simulink model "model_2"  (R2018b)
settings: Solver=FixedStepAuto  StartTime=0.0  StopTime=100  FixedStep=0.0001  MinStep=0.00001  RelTol=1e-5  AbsTol=1e-5
values from neighbouring files (symbols this model uses):
  m = 1    [Drive.m]    (also in on.m)
  N = 1 / T_f    (= 12.8205128205)    [regler.m]
undefined symbols (not defined in the file or in its folder): X, Y, Z
libraries: sm_lib x72, nesl_utility x28, simulink x5, Contact_Forces_Lib x4, simulink_extras x3, vrlib x1
(part 1 of 3)
settings Model: Creator=Crimson  LastModifiedBy=chjal
settings DataIOCC: LimitDataPoints=on
settings OptimizationCC: LifeSpan=inf
settings DebuggingCC: AlgebraicLoopMsg=none  UnconnectedInputMsg=none  UnconnectedOutputMsg=none  UnconnectedLineMsg=none  AllowSymbolicDim=off  SFUnexpectedBacktrackingDiag=warning  SFNoUnconditionalDefaultTransitionDiag=warning  SFExecutionAtInitializationDiag=none
settings SFSimCC: SimUseLocalCustomCode=off
settings RTWCC: RTWUseLocalCustomCode=off
settings CodeAppCC: StateflowObjectComments=on
settings GRTTargetCC: TargetLangStandard=C89/C90 (ANSI)  GeneratePreprocessorConditionals=Disable all
settings ConfigComp: CovMetricSettings=dw  CovHtmlReporting=on  CovSaveCumulativeToWorkspaceVar=on  CovSaveSingleToWorkspaceVar=on  CovExternalEMLEnable=off  CovSFcnEnable=off
settings SimscapeCC: SimscapeNominalValues="[{\"value\":\"10\",\"unit\":\"V\"},{\"value\":\"1\",\"unit\":\"A\"},{\"value\":\"10\",\"unit\":\"N*m\"},{\"value\":\"10\",\"unit\":\"bar\"},{\"value\":\"100\",\"unit\":\"kJ/kg\"},{\"value\":\"1\",\"unit\":\"kW\"},{\"value\":\"300\",\"unit\":\"K\"},{\"value\":\"100\",\"unit\":\"cm^3/s\"},{\"value\":\"1\",\"unit\":\"kN\"},{\"value\":\"1\",\"unit\":\"g/cm^3\"},{\"value\":\"1\",\"unit\":\"l\"},{\"value\":\"1\",\"unit\":\"cm^2\"},{\"value\":\"60\",\"unit\":\"Hz\"}]"  SimscapeLogType=all  SimscapeLogDataHistory=10000
settings ConfigurationSet: Description=SimMechanics 2G
settings DiagnosticsConfigSet: SimMechanicsRigidlyBoundBlock=none

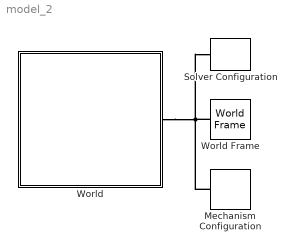
== system model_2 ==
  Mechanism Configuration : sm_lib/Utilities/Mechanism Configuration  UniformGravity=Constant  GravityVector=[0 0 -9.80665]  GravityUnits=m/s^2  LinearizationDelta=0.001
  Solver Configuration : nesl_utility/Solver Configuration  PhysicalDomain=network_engine_domain  SubClassName=solver  LeftPortType=input  RightPortType=generic  Tones=[]  Harmonics=[]  SimulateNoise=off  Profile=off  UseLocalSampling=off  EnableSwitchedLinearOptims=on  FrequencyDomain=off  UseCCode=off  RelTol=0.001  AbsTol=1e-06  MinStep=1e-09  ToWorkspace=off  RevertToSquareIcSolve=off  NumHomotopyIterations=100  PhasorMode=off  PhasorModeNumHarmonics=1  DoDC=off  ResidualTolerance=1e-09  UseLocalSolver=off  LocalSolverChoice=NE_BACKWARD_EULER_ADVANCER  LocalSolverSampleTime=0.001  DoFixedCost=off  MaxNonlinIter=3  MaxModeIter=2  LinearAlgebra=Sparse  EquationFormulation=NE_TIME_EF  DelaysMemoryBudget=1024  AutomaticFiltering=on  FilteringTimeConstant=0.001  PartitionStorageMethod=AS_NEEDED  PartitionMemoryBudget=1024
  World : Subsystem  mask{floorSize=2.5, pathWay=0.5*[-1+0 0-(-3+0.25*tan(2*pi/6)+tan(1*pi/12)+0.5*tan(2*pi/6)); -1+0.5 0-(-3+0.25*tan(2*pi/6)+tan(1*pi/12)+0.5*tan(2*pi/6)); -1+0.5 0.5-(-3+0.25*tan(2*pi/6)+tan(1*pi/12)+0.5*tan(2*pi/6)); -1+1.5 -0.5-(-3+0.25*tan(2*pi/6)+tan(1*pi/12)+0.5*tan(2*pi/6)); -1+1.5 0-(-3+0.25*tan(2*pi/6)+tan(1*pi/12)+0.5*tan(2*pi/6)); -1+2 0-(-3+0.25*tan(2*pi/6)+tan(1*pi/12)+0.5*tan(2*pi/6)); -1+2+cos(5*pi/12) -1+sin(5*pi/12)-(-3+0.25*tan(2*pi/6)+tan(1*pi/12)+0.5*tan(2*pi/6)); -1+2+cos(4*pi/12) -1+sin(4*pi/12)-(-3+0.25*tan(2*pi/6)+tan(1*pi/12)+0.5*tan(2*pi/6)); -1+2+cos(3*pi/12) -1+sin(3*pi/12)-(-3+0.25*tan(2*pi/6)+tan(1*pi/12)+0.5*tan(2*pi/6)); -1+2+cos(2*pi/12) -1+sin(2*pi/12)-(-3+0.25*tan(2*pi/6)+tan(1*pi/12)+0.5*tan(2*pi/6)); -1+2+cos(1*pi/12) -1+sin(1*pi/12)-(-3+0.25*tan(2*pi/6)+tan(1*pi/12)+0.5*tan(2*pi/6)); -1+3 -1-(-3+0.25*tan(2*pi/6)+tan(1*pi/12)+0.5*tan(2*pi/6)); -1+3 -1.5-(-3+0.25*tan(2*pi/6)+tan(1*pi/12)+0.5*tan(2*pi/6)); -1+2.5 -1.75-(-3+0.25*tan(2*pi/6)+tan(1*pi/12)+0.5*tan(2*pi/6)); -1+3.5 -2.25-(-3+0.25*tan(2*pi/6)+tan(1*pi/12)+0.5*tan(2*pi/6)); -1+3 -2.5-(-3+0.25*tan(2*pi/6)+tan(1*pi/12)+0.5*tan(2*pi/6)); -1+3 -3-(-3+0.25*tan(2*pi/6)+tan(1*pi/12)+0.5*tan(2*pi/6)); -1+2.75 -3+0.25*tan(2*pi/6)-(-3+0.25*tan(2*pi/6)+tan(1*pi/12)+0.5*tan(2*pi/6)); -1+0.75 -3+0.25*tan(2*pi/6)-(-3+0.25*tan(2*pi/6)+tan(1*pi/12)+0.5*tan(2*pi/6)); -1+1.75 -3+0.25*tan(2*pi/6)+tan(1*pi/12)-(-3+0.25*tan(2*pi/6)+tan(1*pi/12)+0.5*tan(2*pi/6)); -1+1.25 -3+0.25*tan(2*pi/6)+tan(1*pi/12)+0.5*tan(2*pi/6)-(-3+0.25*tan(2*pi/6)+tan(1*pi/12)+0.5*tan(2*pi/6)); -1+0 -3+0.25*tan(2*pi/6)+tan(1*pi/12)+0.5*tan(2*pi/6)-(-3+0.25*tan(2*pi/6)+tan(1*pi/12)+0.5*tan(2*pi/6)); -1+0 0-(-3+0.25*tan(2*pi/6)+tan(1*pi/12)+0.5*tan(2*pi/6))], floorColor=[1.0 1.0 1.0], floorStiffness=7500, floorDamping=50}
  World Frame : sm_lib/Frames and Transforms/World Frame
  connections:
  Mechanism Configuration/RConn1 -- World/RConn1 -- Solver Configuration/RConn1 -- World Frame/RConn1

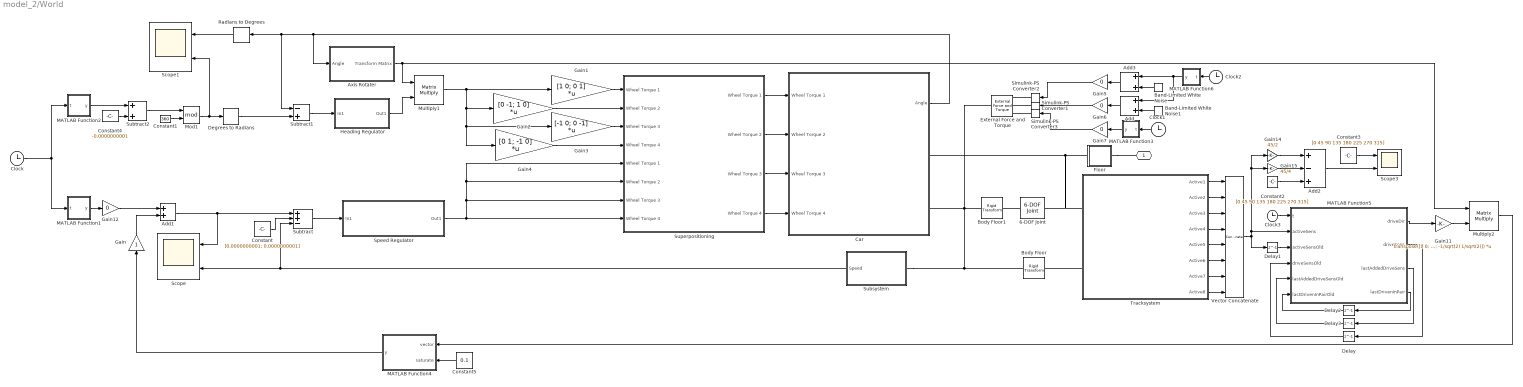
== system model_2/World ==
  6-DOF Joint : sm_lib/Joints/6-DOF Joint  SenseConstraintForce=off  SenseConstraintForceX=off  SenseConstraintForceY=off  SenseConstraintForceZ=off  SenseConstraintTorque=off  SenseConstraintTorqueX=off  SenseConstraintTorqueY=off  SenseConstraintTorqueZ=off  SenseTotalForce=off  SenseTotalForceX=off  SenseTotalForceY=off  SenseTotalForceZ=off  SenseTotalTorque=off  SenseTotalTorqueX=off  SenseTotalTorqueY=off  SenseTotalTorqueZ=off  CompositeWrenchDir=FollowerOnBase  CompositeWrenchFrame=BaseFrame  PxEquilibriumPosition=0  PxEquilibriumPositionUnits=m  PxSpringStiffness=0  PxSpringStiffnessUnits=N/m  PxDampingCoefficient=0  PxDampingCoefficientUnits=N/(m/s)  PxTorqueActuationMode=NoTorque  PxMotionActuationMode=ComputedMotion  PxSensePosition=off  PxSenseVelocity=off  PxSenseAcceleration=off  PxSenseTorqueForce=off  PxPositionTargetSpecify=off  PxPositionTargetPriority=High  PxPositionTargetValue=0  PxPositionTargetValueUnits=m  PxVelocityTargetSpecify=off  PxVelocityTargetPriority=High  PxVelocityTargetValue=0  PxVelocityTargetValueUnits=m/s  PyEquilibriumPosition=0  PyEquilibriumPositionUnits=m  PySpringStiffness=0  PySpringStiffnessUnits=N/m  PyDampingCoefficient=0  PyDampingCoefficientUnits=N/(m/s)  PyTorqueActuationMode=NoTorque  PyMotionActuationMode=ComputedMotion  PySensePosition=off  PySenseVelocity=off  PySenseAcceleration=off  PySenseTorqueForce=off  PyPositionTargetSpecify=off  PyPositionTargetPriority=High  PyPositionTargetValue=0  PyPositionTargetValueUnits=m  PyVelocityTargetSpecify=off  PyVelocityTargetPriority=High  PyVelocityTargetValue=0  PyVelocityTargetValueUnits=m/s  PzEquilibriumPosition=0  PzEquilibriumPositionUnits=m  PzSpringStiffness=0  PzSpringStiffnessUnits=N/m  PzDampingCoefficient=0  PzDampingCoefficientUnits=N/(m/s)  PzTorqueActuationMode=NoTorque  PzMotionActuationMode=ComputedMotion  PzSensePosition=off  PzSenseVelocity=off  PzSenseAcceleration=off  PzSenseTorqueForce=off  PzPositionTargetSpecify=off  PzPositionTargetPriority=High  PzPositionTargetValue=0  PzPositionTargetValueUnits=m  PzVelocityTargetSpecify=off  PzVelocityTargetPriority=High  PzVelocityTargetValue=0  PzVelocityTargetValueUnits=m/s  SphDefPosRotationMethod=None  SphDefPosRotationAngleUnits=deg  SphDefPosRotationStandardAxis=+Z  SphDefPosRotationAngle=0.0  SphDefPosRotationArbitraryAxis=[0 0 1]  SphDefPosFollAlignAxisA=+X  SphDefPosBaseAlignAxisA=+Y  SphDefPosFollAlignAxisB=+Y  SphDefPosBaseAlignAxisB=+Z  SphDefPosRotationSequenceAxes=FollowerAxes  SphDefPosRotationSequence=XYX  SphDefPosRotationSequenceAngles=[0 0 0]  SphDefPosRotationSequenceAnglesUnits=deg  SphDefPosRotationMatrix=[1 0 0; 0 1 0; 0 0 1]  SphEqPosRotationMethod=None  SphEqPosRotationAngleUnits=deg  SphEqPosRotationStandardAxis=+Z  SphEqPosRotationAngle=0.0  SphEqPosRotationArbitraryAxis=[0 0 1]  SphEqPosFollAlignAxisA=+X  SphEqPosBaseAlignAxisA=+Y  SphEqPosFollAlignAxisB=+Y  SphEqPosBaseAlignAxisB=+Z  SphEqPosRotationSequenceAxes=FollowerAxes  SphEqPosRotationSequence=XYX  SphEqPosRotationSequenceAngles=[0 0 0]  SphEqPosRotationSequenceAnglesUnits=deg  SphEqPosRotationMatrix=[1 0 0; 0 1 0; 0 0 1]  SphSpringStiffness=0  SphSpringStiffnessUnits=N*m/deg  SphDampingCoefficient=0  SphDampingCoefficientUnits=N*m/(deg/s)  SphActuateTorqueX=off  SphActuateTorqueY=off  SphActuateTorqueZ=off  SphActuateTorque=off  SphTorqueActuationMode=NoTorque  SphMotionActuationMode=ComputedMotion  SphActuationFrame=BaseFrame  SphSensePosition=off  SphSenseVelocityX=off  SphSenseVelocityY=off  SphSenseVelocityZ=off  SphSenseVelocity=off  SphSenseAccelerationX=off  SphSenseAccelerationY=off  SphSenseAccelerationZ=off  SphSenseAcceleration=off  SphSenseTorqueX=off  SphSenseTorqueY=off  SphSenseTorqueZ=off  SphSenseTorqueForce=off  SphSensingFrame=BaseFrame  SphPositionTargetRotationMethod=None  SphPositionTargetRotationAngleUnits=deg  SphPositionTargetRotationStandardAxis=+Z  SphPositionTargetRotationAngle=0.0  SphPositionTargetRotationArbitraryAxis=[0 0 1]  SphPositionTargetFollAlignAxisA=+X  SphPositionTargetBaseAlignAxisA=+Y  SphPositionTargetFollAlignAxisB=+Y  SphPositionTargetBaseAlignAxisB=+Z  SphPositionTargetRotationSequenceAxes=FollowerAxes  SphPositionTargetRotationSequence=XYX  SphPositionTargetRotationSequenceAngles=[0 0 0]  SphPositionTargetRotationSequenceAnglesUnits=deg  SphPositionTargetRotationMatrix=[1 0 0; 0 1 0; 0 0 1]  SphPositionTargetSpecify=off  SphPositionTargetPriority=High  SphVelocityTargetValue=[0 0 0]  SphVelocityTargetValueUnits=deg/s  SphVelocityTargetSpecify=off  SphVelocityTargetPriority=High  SphVelocityTargetInFollowerFrame=on
  Add : Sum
  Add1 : Sum
  Add2 : Sum  Inputs=+-+
  Add3 : Sum
  Axis Rotater : Subsystem
  Band-Limited White Noise : simulink/Sources/Band-Limited White Noise  Cov=[0.001]  Ts=0.1  seed=[23341]
  Band-Limited White Noise1 : simulink/Sources/Band-Limited White Noise  Cov=[0.001]  Ts=0.1  seed=[23342]
  Body Floor : sm_lib/Frames and Transforms/Rigid Transform  TranslationMethod=None  TranslationStandardOffset=1  TranslationLengthUnit=m  TranslationStandardAxis=-Z  TranslationCartesianOffset=[0 0 0]  TranslationROffset=0  TranslationROffsetUnits=m  TranslationZOffset=0  TranslationZOffsetUnits=m  TranslationThetaOffset=0  TranslationThetaOffsetUnits=deg  RotationMethod=None  RotationAngleUnits=deg  RotationStandardAxis=-Z  RotationAngle=90  RotationArbitraryAxis=[0 0 1]  FollAlignAxisA=+X  BaseAlignAxisA=+Y  FollAlignAxisB=+Y  BaseAlignAxisB=+Z  RotationSequenceAxes=FollowerAxes  RotationSequence=XYX  RotationSequenceAngles=[0 0 0]  RotationSequenceAnglesUnits=deg  RotationMatrix=[1 0 0; 0 1 0; 0 0 1]
  Body Floor1 : sm_lib/Frames and Transforms/Rigid Transform  TranslationMethod=StandardAxis  TranslationStandardOffset=0.25  TranslationLengthUnit=m  TranslationStandardAxis=+X  TranslationCartesianOffset=[0 0 0]  TranslationROffset=0  TranslationROffsetUnits=m  TranslationZOffset=0  TranslationZOffsetUnits=m  TranslationThetaOffset=0  TranslationThetaOffsetUnits=deg  RotationMethod=None  RotationAngleUnits=deg  RotationStandardAxis=-Z  RotationAngle=90  RotationArbitraryAxis=[0 0 1]  FollAlignAxisA=+X  BaseAlignAxisA=+Y  FollAlignAxisB=+Y  BaseAlignAxisB=+Z  RotationSequenceAxes=FollowerAxes  RotationSequence=XYX  RotationSequenceAngles=[0 0 0]  RotationSequenceAnglesUnits=deg  RotationMatrix=[1 0 0; 0 1 0; 0 0 1]
  Car : Subsystem  mask{wheelLengthOffset=120/1000, wheelWidthOffset=100/1000, radius=73/2/1000, angle=0}
  Clock{,1..3} (4 alike) : Clock
  Constant : Constant  Value=[0.0000000001; 0.0000000001]
  Constant1 : Constant  Value=360
  Constant2 : Constant  Value=[0 45 90 135 180 225 270 315]
  Constant3 : Constant  Value=[0 45 90 135 180 225 270 315]
  Constant4 : Constant  Value=-0.0000000001
  Constant5 : Constant  Value=0.1
  Degrees to Radians : simulink_extras/Transformations/Degrees to Radians
  Delay : Delay  DelayLength=1  InitialCondition=[0,0,0,0,1,0,0,0]
  Delay1 : Delay  DelayLength=1  InitialCondition=[1,1,1,1,1,1,1,1]
  Delay2 : Delay  DelayLength=1  InitialCondition=[1,0,0,0,0,0,0,0]
  Delay3 : Delay  DelayLength=1  InitialCondition=[1,0,1,0]
  External Force and Torque : sm_lib/Forces and Torques/External Force and Torque  ForceResolutionFrame=World  EnableForceX=on  EnableForceY=on  EnableForceZ=off  EnableForce=off  TorqueResolutionFrame=World  EnableTorqueX=off  EnableTorqueY=off  EnableTorqueZ=on  EnableTorque=off
  Floor : Subsystem
  Gain : Gain
  Gain1 : Gain  Gain=[1 0; 0 1]  Multiplication=Matrix(K*u)
  Gain11 : Gain  Gain=transpose([1 0; 1/sqrt(2) 1/sqrt(2); 0 1; -1/sqrt(2) 1/sqrt(2)])  Multiplication=Matrix(K*u)
  Gain{5..7,12} (4 alike) : Gain  Gain=0
  Gain14 : Gain  Gain=45/2
  Gain15 : Gain  Gain=45/4
  Gain2 : Gain  Gain=[0 -1; 1 0]  Multiplication=Matrix(K*u)
  Gain3 : Gain  Gain=[-1 0; 0 -1]  Multiplication=Matrix(K*u)
  Gain4 : Gain  Gain=[0 1; -1 0]  Multiplication=Matrix(K*u)
  Heading Regulator : Subsystem
  MATLAB Function1 : MATLAB Function  TreatAsAtomicUnit=on
  MATLAB Function2 : MATLAB Function  TreatAsAtomicUnit=on
  MATLAB Function3 : MATLAB Function  TreatAsAtomicUnit=on
  MATLAB Function4 : MATLAB Function  TreatAsAtomicUnit=on
  MATLAB Function5 : MATLAB Function  TreatAsAtomicUnit=on
  MATLAB Function6 : MATLAB Function  TreatAsAtomicUnit=on
  Mod1 : Math  Operator=mod  SaturateOnIntegerOverflow=on
  Multiply1 : Product  Multiplication=Matrix(*)
  Multiply2 : Product  Multiplication=Matrix(*)
  Radians to Degrees : simulink_extras/Transformations/Radians to Degrees
  Scope : Scope  NumInputPorts=2
  Scope1 : Scope  NumInputPorts=2
  Scope3 : Scope  NumInputPorts=2
  Simulink-PS Converter1 : nesl_utility/Simulink-PS Converter  PhysicalDomain=network_engine_domain  SubClassName=ps_input  LeftPortType=input  RightPortType=output  PseudoPeriodic=off  Frequencies=[]  NoiseDistribution=none  NoiseParameters=[]  Unit=N  AffineConversion=off  FilteringAndDerivatives=provide  SimscapeFilterOrder=1  InputFilterTimeConstant=0.001  UdotUserProvided=0
  Simulink-PS Converter2 : nesl_utility/Simulink-PS Converter  PhysicalDomain=network_engine_domain  SubClassName=ps_input  LeftPortType=input  RightPortType=output  PseudoPeriodic=off  Frequencies=[]  NoiseDistribution=none  NoiseParameters=[]  Unit=N  AffineConversion=off  FilteringAndDerivatives=provide  SimscapeFilterOrder=1  InputFilterTimeConstant=0.001  UdotUserProvided=0
  Simulink-PS Converter3 : nesl_utility/Simulink-PS Converter  PhysicalDomain=network_engine_domain  SubClassName=ps_input  LeftPortType=input  RightPortType=output  PseudoPeriodic=off  Frequencies=[]  NoiseDistribution=none  NoiseParameters=[]  Unit=N*m  AffineConversion=off  FilteringAndDerivatives=provide  SimscapeFilterOrder=1  InputFilterTimeConstant=0.001  UdotUserProvided=0
  Speed Regulator : Subsystem
  Subsystem : Subsystem
  Subtract : Sum  Inputs=++-
  Subtract1 : Sum  Inputs=-+
  Subtract2 : Sum
  Superpositioning : Subsystem
  Tracksystem : Subsystem  InitFcn=run bana2  mask{thickness=50/2000, linePath=0.5*[-1.5+0 0-(-3+0.25*tan(2*pi/6)+tan(1*pi/12)+0.5*tan(2*pi/6)); -1.5+0 -3+0.25*tan(2*pi/6)+tan(1*pi/12)+0.5*tan(2*pi/6)-(-3+0.25*tan(2*pi/6)+tan(1*pi/12)+0.5*tan(2*pi/6)); -1.5+1.25 -3+0.25*tan(2*pi/6)+tan(1*pi/12)+0.5*tan(2*pi/6)-(-3+0.25*tan(2*pi/6)+tan(1*pi/12)+0.5*tan(2*pi/6)); -1.5+1.75 -3+0.25*tan(2*pi/6)+tan(1*pi/12)-(-3+0.25*tan(2*pi/6)+tan(1*pi/12)+0.5*tan(2*pi/6)); -1.5+0.75 -3+0.25*tan(2*pi/6)-(-3+0.25*tan(2*pi/6)+tan(1*pi/12)+0.5*tan(2*pi/6)); -1.5+2.75 -3+0.25*tan(2*pi/6)-(-3+0.25*tan(2*pi/6)+tan(1*pi/12)+0.5*tan(2*pi/6)); -1.5+3 -3-(-3+0.25*tan(2*pi/6)+tan(1*pi/12)+0.5*tan(2*pi/6)); -1.5+3 -2.5-(-3+0.25*tan(2*pi/6)+tan(1*pi/12)+0.5*tan(2*pi/6)); -1.5+3.5 -2.25-(-3+0.25*tan(2*pi/6)+tan(1*pi/12)+0.5*tan(2*pi/6)); -1.5+2.5 -1.75-(-3+0.25*tan(2*pi/6)+tan(1*pi/12)+0.5*tan(2*pi/6)); -1.5+3 -1.5-(-3+0.25*tan(2*pi/6)+tan(1*pi/12)+0.5*tan(2*pi/6)); -1.5+3 -1-(-3+0.25*tan(2*pi/6)+tan(1*pi/12)+0.5*tan(2*pi/6)); -1.5+2+cos(1*pi/12) -1+sin(1*pi/12)-(-3+0.25*tan(2*pi/6)+tan(1*pi/12)+0.5*tan(2*pi/6)); -1.5+2+cos(2*pi/12) -1+sin(2*pi/12)-(-3+0.25*tan(2*pi/6)+tan(1*pi/12)+0.5*tan(2*pi/6)); -1.5+2+cos(3*pi/12) -1+sin(3*pi/12)-(-3+0.25*tan(2*pi/6)+tan(1*pi/12)+0.5*tan(2*pi/6)); -1.5+2+cos(4*pi/12) -1+sin(4*pi/12)-(-3+0.25*tan(2*pi/6)+tan(1*pi/12)+0.5*tan(2*pi/6)); -1.5+2+cos(5*pi/12) -1+sin(5*pi/12)-(-3+0.25*tan(2*pi/6)+tan(1*pi/12)+0.5*tan(2*pi/6)); -1.5+2 0-(-3+0.25*tan(2*pi/6)+tan(1*pi/12)+0.5*tan(2*pi/6)); -1.5+1.5 0-(-3+0.25*tan(2*pi/6)+tan(1*pi/12)+0.5*tan(2*pi/6)); -1.5+1.5 -0.5-(-3+0.25*tan(2*pi/6)+tan(1*pi/12)+0.5*tan(2*pi/6)); -1.5+0.5 0.5-(-3+0.25*tan(2*pi/6)+tan(1*pi/12)+0.5*tan(2*pi/6)); -1.5+0.5 0-(-3+0.25*tan(2*pi/6)+tan(1*pi/12)+0.5*tan(2*pi/6)); -1.5+0 0-(-3+0.25*tan(2*pi/6)+tan(1*pi/12)+0.5*tan(2*pi/6))];, sensorLength=28/1000, sensorWidth=10/1000, sensorHeight=10/1000, sensorRadius=50/1000, sensorSize=5/1000}
      mask prompts: sensorSize "sensorSize (debugging only)"
  Vector Concatenate : Concatenate  NumInputs=8
  " " : PMIOPort  Side=Right
  wires:
  Mod1/1 -> Degrees to Radians/1, Scope1/2
  Constant1/1 -> Mod1/2
  Car/1(Angle) -> Axis Rotater/1(Angle), Radians to Degrees/1, Subtract1/1
  Gain1/1 -> Superpositioning/1(Wheel Torque 1)
  Gain2/1 -> Superpositioning/2(Wheel Torque 2)
  Gain3/1 -> Superpositioning/3(Wheel Torque 3)
  Gain4/1 -> Superpositioning/4(Wheel Torque 4)
  Multiply1/1 -> Gain2/1, Gain4/1, Gain3/1, Gain1/1
  Subtract/1 -> Speed Regulator/1(In1)
  Axis Rotater/1(Transform Matrix) -> Multiply1/1, Multiply2/1
  Subtract1/1 -> Heading Regulator/1(In1)
  Heading Regulator/1(Out1) -> Multiply1/2
  Degrees to Radians/1 -> Subtract1/2
  Radians to Degrees/1 -> Scope1/1
  Constant/1 -> Subtract/2
  MATLAB Function1/1(y) -> Gain12/1
  Gain12/1 -> Add1/1
  MATLAB Function4/1(y) -> Gain/1
  Tracksystem/1(Active1) -> Vector Concatenate/1
  Tracksystem/2(Active2) -> Vector Concatenate/2
  Tracksystem/3(Active3) -> Vector Concatenate/3
  Tracksystem/4(Active4) -> Vector Concatenate/4
  Tracksystem/5(Active5) -> Vector Concatenate/5
  Tracksystem/6(Active6) -> Vector Concatenate/6
  Tracksystem/7(Active7) -> Vector Concatenate/7
  Tracksystem/8(Active8) -> Vector Concatenate/8
  Gain14/1 -> Add2/1
  Constant3/1 -> Scope3/1
  Add2/1 -> Scope3/2
  Constant2/1 -> Add2/3
  Gain15/1 -> Add2/2
  Superpositioning/3(" Wheel Torque 3") -> Car/3(Wheel Torque 3)
  Superpositioning/4(" Wheel Torque 4") -> Car/4(Wheel Torque 4)
  Subtract2/1 -> Mod1/1
  Constant4/1 -> Subtract2/2
  MATLAB Function2/1(y) -> Subtract2/1
  Speed Regulator/1(Out1) -> Superpositioning/5("Wheel Torque 1 "), Superpositioning/6("Wheel Torque 2 "), Superpositioning/7("Wheel Torque 3 "), Superpositioning/8("Wheel Torque 4 ")
  Gain11/1 -> Multiply2/2
  Multiply2/1 -> MATLAB Function4/1(vector)
  Constant5/1 -> MATLAB Function4/2(saturate)
  Vector Concatenate/1 -> MATLAB Function5/2(activeSens), Gain14/1, Gain15/1, Delay1/1
  Delay/1 -> MATLAB Function5/4(driveSensOld)
  MATLAB Function5/1(driveDir) -> Gain11/1
  MATLAB Function5/2(driveSens) -> Delay/1
  Delay1/1 -> MATLAB Function5/3(activeSensOld)
  Add1/1 -> Scope/1, Subtract/1
  Subsystem/1(Speed) -> Scope/2, Subtract/3
  MATLAB Function5/3(lastAddedDriveSens) -> Delay3/1
  Delay3/1 -> MATLAB Function5/5(lastAddedDriveSensOld)
  Gain/1 -> Add1/2
  Superpositioning/2(" Wheel Torque 2") -> Car/2(Wheel Torque 2)
  Clock1/1 -> MATLAB Function3/1(t)
  Gain5/1 -> Simulink-PS Converter2/1
  Gain6/1 -> Simulink-PS Converter1/1
  Gain7/1 -> Simulink-PS Converter3/1
  Clock2/1 -> MATLAB Function6/1(t)
  Clock3/1 -> MATLAB Function5/1(t)
  Clock/1 -> MATLAB Function1/1(t), MATLAB Function2/1(t)
  Add/1 -> Gain6/1
  Add3/1 -> Gain5/1
  MATLAB Function6/1(y) -> Add3/1, Add/1
  Band-Limited White Noise/1 -> Add3/2
  Band-Limited White Noise1/1 -> Add/2
  MATLAB Function3/1(y) -> Gain7/1
  Superpositioning/1(" Wheel Torque 1") -> Car/1(Wheel Torque 1)
  MATLAB Function5/4(lastDrivenInPair) -> Delay2/1
  Delay2/1 -> MATLAB Function5/6(lastDrivenInPairOld)
  connections:
  Floor/RConn1 -- " "/RConn1
  Floor/LConn1 -- Tracksystem/LConn1 -- 6-DOF Joint/RConn1 -- Car/RConn1
  Subsystem/LConn1 -- Body Floor/RConn1 -- Car/RConn2 -- Body Floor1/LConn1 -- External Force and Torque/RConn1
  Tracksystem/LConn2 -- Body Floor/LConn1
  Simulink-PS Converter2/RConn1 -- External Force and Torque/LConn1
  Simulink-PS Converter1/RConn1 -- External Force and Torque/LConn2
  Simulink-PS Converter3/RConn1 -- External Force and Torque/LConn3
  6-DOF Joint/LConn1 -- Body Floor1/RConn1

== system model_2/World/Axis Rotater ==
  Angle : Inport
  MATLAB Function : MATLAB Function  TreatAsAtomicUnit=on
  Transform Matrix : Outport
  wires:
  Angle/1 -> MATLAB Function/1(u)
  MATLAB Function/1(y) -> Transform Matrix/1

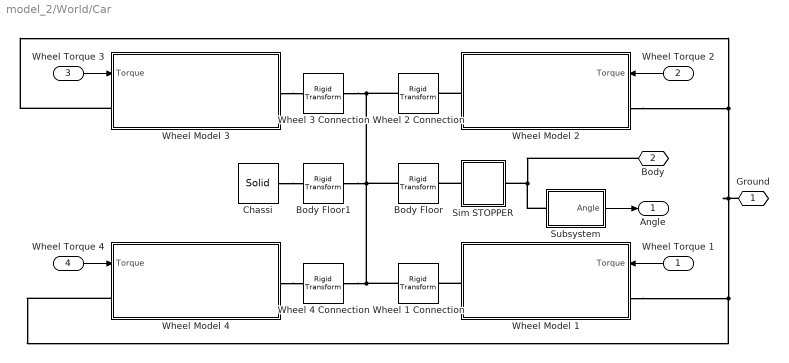
== system model_2/World/Car ==
  Wheel Torque 1 : Inport
  Wheel Torque 2 : Inport  Port=2
  Wheel Torque 3 : Inport  Port=3
  Wheel Torque 4 : Inport  Port=4
  Body Floor : sm_lib/Frames and Transforms/Rigid Transform  TranslationMethod=StandardAxis  TranslationStandardOffset=radius-4.8*10^-4  TranslationLengthUnit=m  TranslationStandardAxis=-Z  TranslationCartesianOffset=[0 0 0]  TranslationROffset=0  TranslationROffsetUnits=m  TranslationZOffset=0  TranslationZOffsetUnits=m  TranslationThetaOffset=0  TranslationThetaOffsetUnits=deg  RotationMethod=StandardAxis  RotationAngleUnits=deg  RotationStandardAxis=-Z  RotationAngle=angle  RotationArbitraryAxis=[0 0 1]  FollAlignAxisA=+X  BaseAlignAxisA=+Y  FollAlignAxisB=+Y  BaseAlignAxisB=+Z  RotationSequenceAxes=FollowerAxes  RotationSequence=XYX  RotationSequenceAngles=[0 0 0]  RotationSequenceAnglesUnits=deg  RotationMatrix=[1 0 0; 0 1 0; 0 0 1]
  Body Floor1 : sm_lib/Frames and Transforms/Rigid Transform  TranslationMethod=Cartesian  TranslationStandardOffset=0  TranslationLengthUnit=m  TranslationStandardAxis=-Z  TranslationCartesianOffset=[wheelLengthOffset wheelWidthOffset 0]  TranslationROffset=0  TranslationROffsetUnits=m  TranslationZOffset=0  TranslationZOffsetUnits=m  TranslationThetaOffset=0  TranslationThetaOffsetUnits=deg  RotationMethod=None  RotationAngleUnits=deg  RotationStandardAxis=+Z  RotationAngle=0.0  RotationArbitraryAxis=[0 0 1]  FollAlignAxisA=+X  BaseAlignAxisA=+Y  FollAlignAxisB=+Y  BaseAlignAxisB=+Z  RotationSequenceAxes=FollowerAxes  RotationSequence=XYX  RotationSequenceAngles=[0 0 0]  RotationSequenceAnglesUnits=deg  RotationMatrix=[1 0 0; 0 1 0; 0 0 1]
  Chassi : sm_lib/Body Elements/Solid  InertiaType=CalculateFromGeometry  Mass=1  MassUnits=kg  CenterOfMass=[0 0 0]  CenterOfMassUnits=m  MomentsOfInertia=[1 1 1]  MomentsOfInertiaUnits=kg*m^2  ProductsOfInertia=[0 0 0]  ProductsOfInertiaUnits=kg*m^2  BasedOnType=Density  Density=2700  DensityUnits=kg/m^3  DoExposeReferenceFrame=on  SerializedFrames=<Frames/>  GraphicType=FromGeometry  MarkerShape=Sphere  MarkerSize=10  GraphicVisPropType=SimpleVisualProperties  GraphicDiffuseColor=[0.6 0.8 1.0]  GraphicSpecularColor=[0.5 0.5 0.5 1.0]  GraphicAmbientColor=[0.15 0.15 0.15 1.0]  GraphicEmissiveColor=[0.0 0.0 0.0 1.0]  GraphicShininess=75  GraphicOpacity=0.5  GeometryShape=FromFile  RectangleSize=[1 1]  RectangleSizeUnits=m  BrickDimensions=[1 1 1]  BrickDimensionUnits=m  CylinderRadius=1  CylinderRadiusUnits=m  CylinderLength=1  CylinderLengthUnits=m  SphereRadius=1  SphereRadiusUnits=m  EllipsoidRadii=[1 1 .5]  EllipsoidRadiiUnits=m  ExtrusionCrossSection=[1 1; -1 1; -1 -1; 1 -1]  ExtrusionCrossSectionUnits=m  ExtrusionLength=1  ExtrusionLengthUnits=m  PolygonNumSides=3  PolygonOuterRadius=1  PolygonOuterRadiusUnits=m  ExtGeomFileType=STEP  ExtGeomFileName=bas.stp  ExtGeomFileUnits=m  RevolutionCrossSection=[1 1; 1 -1; 2 -1; 2 1]  RevolutionCrossSectionUnits=m  RevolutionExtent=Custom  RevolutionAngle=180  RevolutionAngleUnits=deg
  Sim STOPPER : Subsystem
  Subsystem : Subsystem
  Wheel 1 Connection : sm_lib/Frames and Transforms/Rigid Transform  TranslationMethod=Cartesian  TranslationStandardOffset=1  TranslationLengthUnit=m  TranslationStandardAxis=-Z  TranslationCartesianOffset=[wheelLengthOffset -wheelWidthOffset 0]  TranslationROffset=0  TranslationROffsetUnits=m  TranslationZOffset=0  TranslationZOffsetUnits=m  TranslationThetaOffset=0  TranslationThetaOffsetUnits=deg  RotationMethod=StandardAxis  RotationAngleUnits=deg  RotationStandardAxis=+Z  RotationAngle=180  RotationArbitraryAxis=[0 0 1]  FollAlignAxisA=+X  BaseAlignAxisA=+Y  FollAlignAxisB=+Y  BaseAlignAxisB=+Z  RotationSequenceAxes=FollowerAxes  RotationSequence=XYX  RotationSequenceAngles=[0 0 0]  RotationSequenceAnglesUnits=deg  RotationMatrix=[1 0 0; 0 1 0; 0 0 1]
  Wheel 2 Connection : sm_lib/Frames and Transforms/Rigid Transform  TranslationMethod=Cartesian  TranslationStandardOffset=0  TranslationLengthUnit=m  TranslationStandardAxis=-Z  TranslationCartesianOffset=[wheelLengthOffset wheelWidthOffset 0]  TranslationROffset=0  TranslationROffsetUnits=m  TranslationZOffset=0  TranslationZOffsetUnits=m  TranslationThetaOffset=0  TranslationThetaOffsetUnits=deg  RotationMethod=StandardAxis  RotationAngleUnits=deg  RotationStandardAxis=+Z  RotationAngle=0.0  RotationArbitraryAxis=[0 0 1]  FollAlignAxisA=+X  BaseAlignAxisA=+Y  FollAlignAxisB=+Y  BaseAlignAxisB=+Z  RotationSequenceAxes=FollowerAxes  RotationSequence=XYX  RotationSequenceAngles=[0 0 0]  RotationSequenceAnglesUnits=deg  RotationMatrix=[1 0 0; 0 1 0; 0 0 1]
  Wheel 3 Connection : sm_lib/Frames and Transforms/Rigid Transform  TranslationMethod=Cartesian  TranslationStandardOffset=0  TranslationLengthUnit=m  TranslationStandardAxis=-Z  TranslationCartesianOffset=[-wheelLengthOffset wheelWidthOffset 0]  TranslationROffset=0  TranslationROffsetUnits=m  TranslationZOffset=0  TranslationZOffsetUnits=m  TranslationThetaOffset=0  TranslationThetaOffsetUnits=deg  RotationMethod=StandardAxis  RotationAngleUnits=deg  RotationStandardAxis=+Z  RotationAngle=0.0  RotationArbitraryAxis=[0 0 1]  FollAlignAxisA=+X  BaseAlignAxisA=+Y  FollAlignAxisB=+Y  BaseAlignAxisB=+Z  RotationSequenceAxes=FollowerAxes  RotationSequence=XYX  RotationSequenceAngles=[0 0 0]  RotationSequenceAnglesUnits=deg  RotationMatrix=[1 0 0; 0 1 0; 0 0 1]
  Wheel 4 Connection : sm_lib/Frames and Transforms/Rigid Transform  TranslationMethod=Cartesian  TranslationStandardOffset=0  TranslationLengthUnit=m  TranslationStandardAxis=-Z  TranslationCartesianOffset=[-wheelLengthOffset -wheelWidthOffset 0]  TranslationROffset=0  TranslationROffsetUnits=m  TranslationZOffset=0  TranslationZOffsetUnits=m  TranslationThetaOffset=0  TranslationThetaOffsetUnits=deg  RotationMethod=StandardAxis  RotationAngleUnits=deg  RotationStandardAxis=+Z  RotationAngle=180  RotationArbitraryAxis=[0 0 1]  FollAlignAxisA=+X  BaseAlignAxisA=+Y  FollAlignAxisB=+Y  BaseAlignAxisB=+Z  RotationSequenceAxes=FollowerAxes  RotationSequence=XYX  RotationSequenceAngles=[0 0 0]  RotationSequenceAnglesUnits=deg  RotationMatrix=[1 0 0; 0 1 0; 0 0 1]
  Wheel Model 1 : Subsystem
  Wheel Model 2 : Subsystem
  Wheel Model 3 : Subsystem
  Wheel Model 4 : Subsystem
  Ground : PMIOPort  Side=Right
  Body : PMIOPort  Port=2  Side=Right
  Angle : Outport
  wires:
  Wheel Torque 2/1 -> Wheel Model 2/1(Torque)
  Wheel Torque 3/1 -> Wheel Model 3/1(Torque)
  Subsystem/1(Angle) -> Angle/1
  Wheel Torque 1/1 -> Wheel Model 1/1(Torque)
  Wheel Torque 4/1 -> Wheel Model 4/1(Torque)
  connections:
  Wheel 2 Connection/LConn1 -- Wheel 4 Connection/LConn1 -- Wheel 1 Connection/LConn1 -- Body Floor1/RConn1 -- Body Floor/LConn1 -- Wheel 3 Connection/LConn1
  Subsystem/LConn1 -- Body/RConn1 -- Sim STOPPER/RConn1
  Wheel Model 3/RConn1 -- Wheel 3 Connection/RConn1
  Chassi/RConn1 -- Body Floor1/LConn1
  Wheel Model 2/RConn1 -- Wheel 2 Connection/RConn1
  Sim STOPPER/LConn1 -- Body Floor/RConn1
  Ground/RConn1 -- Wheel Model 3/LConn1 -- Wheel Model 2/LConn1 -- Wheel Model 4/LConn1 -- Wheel Model 1/LConn1
  Wheel Model 1/RConn1 -- Wheel 1 Connection/RConn1
  Wheel Model 4/RConn1 -- Wheel 4 Connection/RConn1

== system model_2/World/Floor ==
  Floor : sm_lib/Body Elements/Solid  InertiaType=CalculateFromGeometry  Mass=1  MassUnits=kg  CenterOfMass=[0 0 0]  CenterOfMassUnits=m  MomentsOfInertia=[1 1 1]  MomentsOfInertiaUnits=kg*m^2  ProductsOfInertia=[0 0 0]  ProductsOfInertiaUnits=kg*m^2  BasedOnType=Density  Density=1000  DensityUnits=kg/(m^3)  DoExposeReferenceFrame=on  SerializedFrames=<Frames/>  GraphicType=FromGeometry  MarkerShape=Cube  MarkerSize=5000  GraphicVisPropType=SimpleVisualProperties  GraphicDiffuseColor=floorColor  GraphicSpecularColor=[0.5 0.5 0.5 1.0]  GraphicAmbientColor=[0.15 0.15 0.15 1.0]  GraphicEmissiveColor=[0.0 0.0 0.0 1.0]  GraphicShininess=75  GraphicOpacity=1.0  GeometryShape=Brick  RectangleSize=[1 1]  RectangleSizeUnits=m  BrickDimensions=[floorSize floorSize, floorSize/1000]  BrickDimensionUnits=m  CylinderRadius=1  CylinderRadiusUnits=m  CylinderLength=1  CylinderLengthUnits=m  SphereRadius=1  SphereRadiusUnits=m  EllipsoidRadii=[1 1 1]  EllipsoidRadiiUnits=m  ExtrusionCrossSection=[1 1; -1 1; -1 -1; 1 -1]  ExtrusionCrossSectionUnits=m  ExtrusionLength=floorSize/1000  ExtrusionLengthUnits=m  PolygonNumSides=3  PolygonOuterRadius=1  PolygonOuterRadiusUnits=m  ExtGeomFileType=STL  ExtGeomFileUnits=m  RevolutionCrossSection=[1 1; 1 -1; 2 -1; 2 1]  RevolutionCrossSectionUnits=m  RevolutionExtent=Full  RevolutionAngle=180  RevolutionAngleUnits=deg
  Floor Surface : sm_lib/Frames and Transforms/Rigid Transform  TranslationMethod=StandardAxis  TranslationStandardOffset=floorSize/2000  TranslationLengthUnit=m  TranslationStandardAxis=+Z  TranslationCartesianOffset=[0 0 0]  TranslationROffset=0  TranslationROffsetUnits=m  TranslationZOffset=0  TranslationZOffsetUnits=m  TranslationThetaOffset=0  TranslationThetaOffsetUnits=deg  RotationMethod=None  RotationAngleUnits=deg  RotationStandardAxis=+Z  RotationAngle=0.0  RotationArbitraryAxis=[0 0 1]  FollAlignAxisA=+X  BaseAlignAxisA=+Y  FollAlignAxisB=+Y  BaseAlignAxisB=+Z  RotationSequenceAxes=FollowerAxes  RotationSequence=XYX  RotationSequenceAngles=[0 0 0]  RotationSequenceAnglesUnits=deg  RotationMatrix=[1 0 0; 0 1 0; 0 0 1]
  " " : PMIOPort  Side=Left
  " " : PMIOPort  Port=2  Side=Right
  connections:
  Floor/RConn1 -- Floor Surface/LConn1
  Floor Surface/RConn1 -- " "/RConn1

== system model_2/World/Heading Regulator ==
  In1 : Inport
  Constant3 : Constant  Value=[100/1000; 120/1000]
  MATLAB Function : MATLAB Function  TreatAsAtomicUnit=on
  Normalize Vector : vrlib/Utilities/Normalize Vector  maxzero=0
      settings: SourceProductName=Simulink 3D Animation  SourceProductBaseCode=VR
  PID Controller1 : simulink/Continuous/PID Controller  Controller=PID  Form=Parallel  TimeDomain=Continuous-time  SampleTime=-1  IntegratorMethod=Forward Euler  FilterMethod=Forward Euler  ControllerParametersSource=internal  P=0.027  I=0.026  D=0.01326  UseFilter=on  N=12.82  TunerSelectOption=Transfer Function Based (PID Tuner App)  InitialConditionSource=internal  InitialConditionForIntegrator=0  InitialConditionForFilter=0  DifferentiatorICPrevScaledInput=0  ExternalReset=none  TrackingMode=off  Kt=1  LimitOutput=off  UpperSaturationLimit=inf  LowerSaturationLimit=-inf  LinearizeAsGain=on  AntiWindupMode=none  Kb=1  POutMin=[]  POutMax=[]  IOutMin=[]  IOutMax=[]  DOutMin=[]  DOutMax=[]  NOutMin=[]  NOutMax=[]  SumOutMin=[]  SumOutMax=[]  SaturationOutMin=[]  SaturationOutMax=[]  PParamMin=[]  PParamMax=[]  IParamMin=[]  IParamMax=[]  DParamMin=[]  DParamMax=[]  NParamMin=[]  NParamMax=[]  KbParamMin=[]  KbParamMax=[]  KtParamMin=[]  KtParamMax=[]  KbOutMin=[]  KbOutMax=[]  KtOutMin=[]  KtOutMax=[]  IntegratorOutMin=[]  IntegratorOutMax=[]  FilterOutMin=[]  FilterOutMax=[]  SumI1OutMin=[]  SumI1OutMax=[]  SumI2OutMin=[]  SumI2OutMax=[]  SumI3OutMin=[]  SumI3OutMax=[]  SumI4OutMin=[]  SumI4OutMax=[]  SumDOutMin=[]  SumDOutMax=[]  DifferentiatorOutMin=[]  DifferentiatorOutMax=[]  FilterDiffOutCoefMin=[]  FilterDiffOutCoefMax=[]  ReciprocalOutMin=[]  ReciprocalOutMax=[]  SumDenOutMin=[]  SumDenOutMax=[]  SumNumOutMin=[]  SumNumOutMax=[]  DivideOutMin=[]  DivideOutMax=[]  IntegratorContinuousStateAttributes=''  IntegratorStateMustResolveToSignalObject=off  IntegratorRTWStateStorageClass=Auto  FilterContinuousStateAttributes=''  FilterStateMustResolveToSignalObject=off  FilterRTWStateStorageClass=Auto  ParallelPVariant=InternalParameters  IdealPVariant=Disabled  IVariant=InternalParameters  DVariant=InternalParameters  IntegratorVariant=Continuous  SatVariant=Disabled  AWVariant=Passthrough  PCopyVariant=Disabled  TRVariant=Disabled  FdbkBlocksVariant=Forward  IdealPFdbkVariant=Disabled  SatFdbkVariant=Disabled  DerivativeFilterVariant=ContFilter  NVariant=InternalParameters  NCopyVariant=Disabled  FilterICVariant=InternalICsFilter  IntegratorICVariant=InternalICs  ExternalResetVariant=Disabled  TRSumVariant=Passthrough  SumFdbkVariant=Disabled  SumVariant=Sum_PID
  Product : Product
  Scope : Scope
  Out1 : Outport
  wires:
  In1/1 -> MATLAB Function/1(u)
  Constant3/1 -> Normalize Vector/1
  MATLAB Function/1(y) -> PID Controller1/1
  Product/1 -> Out1/1
  Normalize Vector/1 -> Product/1
  PID Controller1/1 -> Scope/1, Product/2

== system model_2/World/Speed Regulator ==
  In1 : Inport
  PID Controller1 : simulink/Continuous/PID Controller  Controller=PID  Form=Parallel  TimeDomain=Continuous-time  SampleTime=-1  IntegratorMethod=Forward Euler  FilterMethod=Forward Euler  ControllerParametersSource=internal  P=0.12  I=0.063  D=0  UseFilter=on  N=100  TunerSelectOption=Transfer Function Based (PID Tuner App)  InitialConditionSource=internal  InitialConditionForIntegrator=0  InitialConditionForFilter=0  DifferentiatorICPrevScaledInput=0  ExternalReset=none  TrackingMode=off  Kt=1  LimitOutput=off  UpperSaturationLimit=inf  LowerSaturationLimit=-inf  LinearizeAsGain=on  AntiWindupMode=none  Kb=1  POutMin=[]  POutMax=[]  IOutMin=[]  IOutMax=[]  DOutMin=[]  DOutMax=[]  NOutMin=[]  NOutMax=[]  SumOutMin=[]  SumOutMax=[]  SaturationOutMin=[]  SaturationOutMax=[]  PParamMin=[]  PParamMax=[]  IParamMin=[]  IParamMax=[]  DParamMin=[]  DParamMax=[]  NParamMin=[]  NParamMax=[]  KbParamMin=[]  KbParamMax=[]  KtParamMin=[]  KtParamMax=[]  KbOutMin=[]  KbOutMax=[]  KtOutMin=[]  KtOutMax=[]  IntegratorOutMin=[]  IntegratorOutMax=[]  FilterOutMin=[]  FilterOutMax=[]  SumI1OutMin=[]  SumI1OutMax=[]  SumI2OutMin=[]  SumI2OutMax=[]  SumI3OutMin=[]  SumI3OutMax=[]  SumI4OutMin=[]  SumI4OutMax=[]  SumDOutMin=[]  SumDOutMax=[]  DifferentiatorOutMin=[]  DifferentiatorOutMax=[]  FilterDiffOutCoefMin=[]  FilterDiffOutCoefMax=[]  ReciprocalOutMin=[]  ReciprocalOutMax=[]  SumDenOutMin=[]  SumDenOutMax=[]  SumNumOutMin=[]  SumNumOutMax=[]  DivideOutMin=[]  DivideOutMax=[]  IntegratorContinuousStateAttributes=''  IntegratorStateMustResolveToSignalObject=off  IntegratorRTWStateStorageClass=Auto  FilterContinuousStateAttributes=''  FilterStateMustResolveToSignalObject=off  FilterRTWStateStorageClass=Auto  ParallelPVariant=InternalParameters  IdealPVariant=Disabled  IVariant=InternalParameters  DVariant=InternalParameters  IntegratorVariant=Continuous  SatVariant=Disabled  AWVariant=Passthrough  PCopyVariant=Disabled  TRVariant=Disabled  FdbkBlocksVariant=Forward  IdealPFdbkVariant=Disabled  SatFdbkVariant=Disabled  DerivativeFilterVariant=ContFilter  NVariant=InternalParameters  NCopyVariant=Disabled  FilterICVariant=InternalICsFilter  IntegratorICVariant=InternalICs  ExternalResetVariant=Disabled  TRSumVariant=Passthrough  SumFdbkVariant=Disabled  SumVariant=Sum_PID
  Out1 : Outport
  wires:
  PID Controller1/1 -> Out1/1
  In1/1 -> PID Controller1/1

== system model_2/World/Subsystem ==
  Gain3 : Gain  Gain=-1
  PS-Simulink Converter : nesl_utility/PS-Simulink Converter  PhysicalDomain=network_engine_domain  SubClassName=ps_output  LeftPortType=input  RightPortType=output  PseudoPeriodic=off  Frequencies=[]  Unit=1  AffineConversion=off
  PS-Simulink Converter1 : nesl_utility/PS-Simulink Converter  PhysicalDomain=network_engine_domain  SubClassName=ps_output  LeftPortType=input  RightPortType=output  PseudoPeriodic=off  Frequencies=[]  Unit=1  AffineConversion=off
  Transform Sensor : sm_lib/Frames and Transforms/Transform Sensor  MeasurementFrame=World  SenseAngle=off  SenseAxis=off  SenseAngle1=off  SenseAngle2=off  SenseAngle3=off  SenseQ=off  SenseR=off  SenseOmegaX=off  SenseOmegaY=off  SenseOmegaZ=off  SenseOmega1=off  SenseOmega2=off  SenseOmega3=off  SenseQDot=off  SenseRDot=off  SenseAlphaX=off  SenseAlphaY=off  SenseAlphaZ=off  SenseAlpha1=off  SenseAlpha2=off  SenseAlpha3=off  SenseQDDot=off  SenseRDDot=off  SenseX=off  SenseY=off  SenseZ=off  SenseRad=off  SenseAzim=off  SenseDist=off  SenseInc=off  SenseXDot=on  SenseYDot=on  SenseZDot=off  SenseRadDot=off  SenseAzimDot=off  SenseDistDot=off  SenseIncDot=off  SenseXDDot=off  SenseYDDot=off  SenseZDDot=off  SenseRadDDot=off  SenseAzimDDot=off  SenseDistDDot=off  SenseIncDDot=off
  Vector Concatenate : Concatenate
  Body : PMIOPort  Side=Left
  Speed : Outport
  wires:
  PS-Simulink Converter/1 -> Vector Concatenate/1
  Vector Concatenate/1 -> Gain3/1
  PS-Simulink Converter1/1 -> Vector Concatenate/2
  Gain3/1 -> Speed/1
  connections:
  PS-Simulink Converter1/LConn1 -- Transform Sensor/RConn3
  PS-Simulink Converter/LConn1 -- Transform Sensor/RConn2
  Transform Sensor/LConn1 -- Body/RConn1

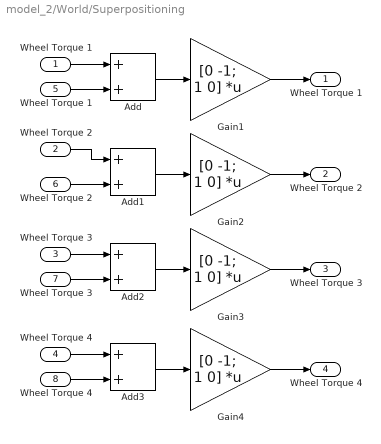
== system model_2/World/Superpositioning ==
  Wheel Torque 1 : Inport
  Wheel Torque 2 : Inport  Port=2
  Wheel Torque 3 : Inport  Port=3
  Wheel Torque 4 : Inport  Port=4
  "Wheel Torque 1 " : Inport  Port=5
  "Wheel Torque 2 " : Inport  Port=6
  "Wheel Torque 3 " : Inport  Port=7
  "Wheel Torque 4 " : Inport  Port=8
  Add{,1..3} (4 alike) : Sum
  Gain{1..4} (4 alike) : Gain  Gain=[0 -1; 1 0]  Multiplication=Matrix(K*u)
  " Wheel Torque 1" : Outport
  " Wheel Torque 2" : Outport  Port=2
  " Wheel Torque 3" : Outport  Port=3
  " Wheel Torque 4" : Outport  Port=4
  wires:
  Add/1 -> Gain1/1
  Wheel Torque 1/1 -> Add/1
  "Wheel Torque 1 "/1 -> Add/2
  Add1/1 -> Gain2/1
  Wheel Torque 2/1 -> Add1/1
  "Wheel Torque 2 "/1 -> Add1/2
  Add2/1 -> Gain3/1
  Wheel Torque 3/1 -> Add2/1
  "Wheel Torque 3 "/1 -> Add2/2
  Add3/1 -> Gain4/1
  Wheel Torque 4/1 -> Add3/1
  "Wheel Torque 4 "/1 -> Add3/2
  Gain1/1 -> " Wheel Torque 1"/1
  Gain2/1 -> " Wheel Torque 2"/1
  Gain3/1 -> " Wheel Torque 3"/1
  Gain4/1 -> " Wheel Torque 4"/1

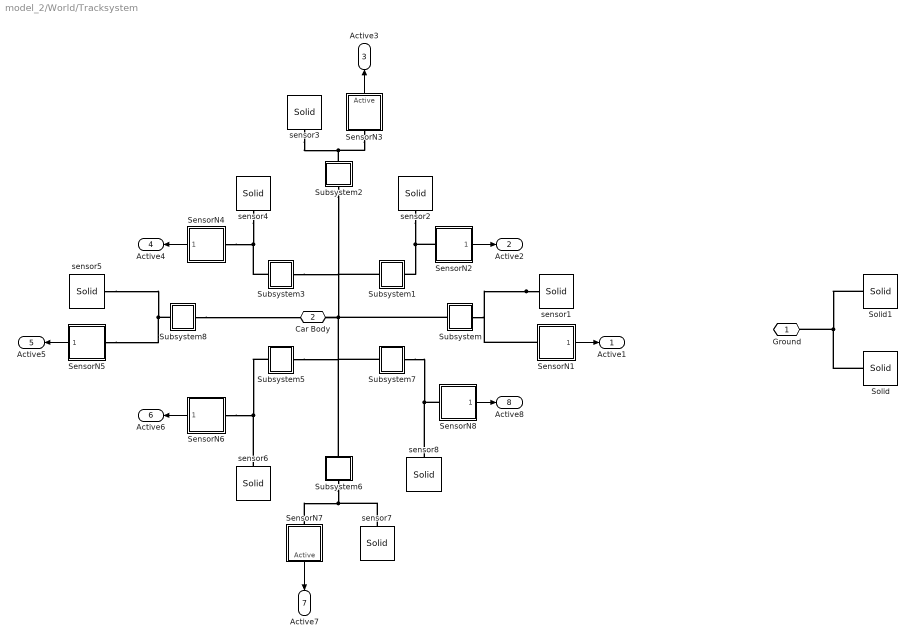
== system model_2/World/Tracksystem ==
  SensorN1 : Subsystem
  SensorN2 : Subsystem
  SensorN3 : Subsystem
  SensorN4 : Subsystem
  SensorN5 : Subsystem
  SensorN6 : Subsystem
  SensorN7 : Subsystem
  SensorN8 : Subsystem
  Solid : sm_lib/Body Elements/Solid  InertiaType=CalculateFromGeometry  Mass=1  MassUnits=kg  CenterOfMass=[0 0 0]  CenterOfMassUnits=m  MomentsOfInertia=[1 1 1]  MomentsOfInertiaUnits=kg*m^2  ProductsOfInertia=[0 0 0]  ProductsOfInertiaUnits=kg*m^2  BasedOnType=Density  Density=1000  DensityUnits=kg/m^3  DoExposeReferenceFrame=on  SerializedFrames=<Frames/>  GraphicType=FromGeometry  MarkerShape=Sphere  MarkerSize=10  GraphicVisPropType=SimpleVisualProperties  GraphicDiffuseColor=[0.5 0.5 0.5]  GraphicSpecularColor=[0.5 0.5 0.5 1.0]  GraphicAmbientColor=[0.15 0.15 0.15 1.0]  GraphicEmissiveColor=[0.0 0.0 0.0 1.0]  GraphicShininess=75  GraphicOpacity=1.0  GeometryShape=GeneralExtrusion  RectangleSize=[1 1]  RectangleSizeUnits=m  BrickDimensions=[1 1 1]  BrickDimensionUnits=m  CylinderRadius=1  CylinderRadiusUnits=m  CylinderLength=1  CylinderLengthUnits=m  SphereRadius=1  SphereRadiusUnits=m  EllipsoidRadii=[1 1 1]  EllipsoidRadiiUnits=m  ExtrusionCrossSection=OuterLines  ExtrusionCrossSectionUnits=m  ExtrusionLength=floorSize/200000  ExtrusionLengthUnits=m  PolygonNumSides=3  PolygonOuterRadius=1  PolygonOuterRadiusUnits=m  ExtGeomFileType=STEP  ExtGeomFileUnits=m  RevolutionCrossSection=[1 1; 1 -1; 2 -1; 2 1]  RevolutionCrossSectionUnits=m  RevolutionExtent=Full  RevolutionAngle=180  RevolutionAngleUnits=deg
  Solid1 : sm_lib/Body Elements/Solid  InertiaType=CalculateFromGeometry  Mass=1  MassUnits=kg  CenterOfMass=[0 0 0]  CenterOfMassUnits=m  MomentsOfInertia=[1 1 1]  MomentsOfInertiaUnits=kg*m^2  ProductsOfInertia=[0 0 0]  ProductsOfInertiaUnits=kg*m^2  BasedOnType=Density  Density=1000  DensityUnits=kg/m^3  DoExposeReferenceFrame=on  SerializedFrames=<Frames/>  GraphicType=FromGeometry  MarkerShape=Sphere  MarkerSize=10  GraphicVisPropType=SimpleVisualProperties  GraphicDiffuseColor=floorColor  GraphicSpecularColor=[0.5 0.5 0.5 1.0]  GraphicAmbientColor=[0.15 0.15 0.15 1.0]  GraphicEmissiveColor=[0.0 0.0 0.0 1.0]  GraphicShininess=75  GraphicOpacity=1.0  GeometryShape=GeneralExtrusion  RectangleSize=[1 1]  RectangleSizeUnits=m  BrickDimensions=[1 1 1]  BrickDimensionUnits=m  CylinderRadius=1  CylinderRadiusUnits=m  CylinderLength=1  CylinderLengthUnits=m  SphereRadius=1  SphereRadiusUnits=m  EllipsoidRadii=[1 1 1]  EllipsoidRadiiUnits=m  ExtrusionCrossSection=InnerLines  ExtrusionCrossSectionUnits=m  ExtrusionLength=floorSize/100000  ExtrusionLengthUnits=m  PolygonNumSides=3  PolygonOuterRadius=1  PolygonOuterRadiusUnits=m  ExtGeomFileType=STEP  ExtGeomFileUnits=m  RevolutionCrossSection=[1 1; 1 -1; 2 -1; 2 1]  RevolutionCrossSectionUnits=m  RevolutionExtent=Full  RevolutionAngle=180  RevolutionAngleUnits=deg
  Subsystem : Subsystem  mask{angle=0}
  Subsystem1 : Subsystem  mask{angle=45}
  Subsystem2 : Subsystem  mask{angle=90}
  Subsystem3 : Subsystem  mask{angle=90+45}
  Subsystem5 : Subsystem  mask{angle=180+45}
  Subsystem6 : Subsystem  mask{angle=270}
  Subsystem7 : Subsystem  mask{angle=270+45}
  Subsystem8 : Subsystem  mask{angle=180}
  sensor{1,5..8} (5 alike) : sm_lib/Body Elements/Solid  InertiaType=CalculateFromGeometry  Mass=1/1000  MassUnits=kg  CenterOfMass=[0 0 0]  CenterOfMassUnits=m  MomentsOfInertia=[1 1 1]  MomentsOfInertiaUnits=kg*m^2  ProductsOfInertia=[0 0 0]  ProductsOfInertiaUnits=kg*m^2  BasedOnType=Mass  Density=1000  DensityUnits=kg/m^3  DoExposeReferenceFrame=on  SerializedFrames=<Frames/>  GraphicType=FromGeometry  MarkerShape=Sphere  MarkerSize=10  GraphicVisPropType=SimpleVisualProperties  GraphicDiffuseColor=[1.0 1.0 0.2]  GraphicSpecularColor=[0.5 0.5 0.5 1.0]  GraphicAmbientColor=[0.15 0.15 0.15 1.0]  GraphicEmissiveColor=[0.0 0.0 0.0 1.0]  GraphicShininess=75  GraphicOpacity=1.0  GeometryShape=Cylinder  RectangleSize=[1 1]  RectangleSizeUnits=m  BrickDimensions=[sensorLength sensorWidth sensorHeight]  BrickDimensionUnits=m  CylinderRadius=sensorSize  CylinderRadiusUnits=m  CylinderLength=sensorHeight  CylinderLengthUnits=m  SphereRadius=1  SphereRadiusUnits=m  EllipsoidRadii=[1 1 .5]  EllipsoidRadiiUnits=m  ExtrusionCrossSection=[1 1; -1 1; -1 -1; 1 -1]  ExtrusionCrossSectionUnits=m  ExtrusionLength=1  ExtrusionLengthUnits=m  PolygonNumSides=3  PolygonOuterRadius=1  PolygonOuterRadiusUnits=m  ExtGeomFileType=STEP  ExtGeomFileName=Bas_assembly_v2.stp  ExtGeomFileUnits=m  RevolutionCrossSection=[1 1; 1 -1; 2 -1; 2 1]  RevolutionCrossSectionUnits=m  RevolutionExtent=Custom  RevolutionAngle=180  RevolutionAngleUnits=deg
  sensor2 : sm_lib/Body Elements/Solid  InertiaType=CalculateFromGeometry  Mass=1/1000  MassUnits=kg  CenterOfMass=[0 0 0]  CenterOfMassUnits=m  MomentsOfInertia=[1 1 1]  MomentsOfInertiaUnits=kg*m^2  ProductsOfInertia=[0 0 0]  ProductsOfInertiaUnits=kg*m^2  BasedOnType=Mass  Density=1/1000  DensityUnits=kg/m^3  DoExposeReferenceFrame=on  SerializedFrames=<Frames/>  GraphicType=FromGeometry  MarkerShape=Sphere  MarkerSize=10  GraphicVisPropType=SimpleVisualProperties  GraphicDiffuseColor=[1.0 1.0 0.2]  GraphicSpecularColor=[0.5 0.5 0.5 1.0]  GraphicAmbientColor=[0.15 0.15 0.15 1.0]  GraphicEmissiveColor=[0.0 0.0 0.0 1.0]  GraphicShininess=75  GraphicOpacity=1.0  GeometryShape=Cylinder  RectangleSize=[1 1]  RectangleSizeUnits=m  BrickDimensions=[sensorLength sensorWidth sensorHeight]  BrickDimensionUnits=m  CylinderRadius=sensorSize  CylinderRadiusUnits=m  CylinderLength=sensorHeight  CylinderLengthUnits=m  SphereRadius=1  SphereRadiusUnits=m  EllipsoidRadii=[1 1 .5]  EllipsoidRadiiUnits=m  ExtrusionCrossSection=[1 1; -1 1; -1 -1; 1 -1]  ExtrusionCrossSectionUnits=m  ExtrusionLength=1  ExtrusionLengthUnits=m  PolygonNumSides=3  PolygonOuterRadius=1  PolygonOuterRadiusUnits=m  ExtGeomFileType=STEP  ExtGeomFileName=Bas_assembly_v2.stp  ExtGeomFileUnits=m  RevolutionCrossSection=[1 1; 1 -1; 2 -1; 2 1]  RevolutionCrossSectionUnits=m  RevolutionExtent=Custom  RevolutionAngle=180  RevolutionAngleUnits=deg
  sensor3 : sm_lib/Body Elements/Solid  InertiaType=CalculateFromGeometry  Mass=1/1000  MassUnits=kg  CenterOfMass=[0 0 0]  CenterOfMassUnits=m  MomentsOfInertia=[1 1 1]  MomentsOfInertiaUnits=kg*m^2  ProductsOfInertia=[0 0 0]  ProductsOfInertiaUnits=kg*m^2  BasedOnType=Mass  Density=1/1000  DensityUnits=kg/m^3  DoExposeReferenceFrame=on  SerializedFrames=<Frames/>  GraphicType=FromGeometry  MarkerShape=Sphere  MarkerSize=10  GraphicVisPropType=SimpleVisualProperties  GraphicDiffuseColor=[1.0 1.0 0.2]  GraphicSpecularColor=[0.5 0.5 0.5 1.0]  GraphicAmbientColor=[0.15 0.15 0.15 1.0]  GraphicEmissiveColor=[0.0 0.0 0.0 1.0]  GraphicShininess=75  GraphicOpacity=1.0  GeometryShape=Cylinder  RectangleSize=[1 1]  RectangleSizeUnits=m  BrickDimensions=[sensorLength sensorWidth sensorHeight]  BrickDimensionUnits=m  CylinderRadius=sensorSize  CylinderRadiusUnits=m  CylinderLength=sensorHeight  CylinderLengthUnits=m  SphereRadius=1  SphereRadiusUnits=m  EllipsoidRadii=[1 1 .5]  EllipsoidRadiiUnits=m  ExtrusionCrossSection=[1 1; -1 1; -1 -1; 1 -1]  ExtrusionCrossSectionUnits=m  ExtrusionLength=1  ExtrusionLengthUnits=m  PolygonNumSides=3  PolygonOuterRadius=1  PolygonOuterRadiusUnits=m  ExtGeomFileType=STEP  ExtGeomFileName=Bas_assembly_v2.stp  ExtGeomFileUnits=m  RevolutionCrossSection=[1 1; 1 -1; 2 -1; 2 1]  RevolutionCrossSectionUnits=m  RevolutionExtent=Custom  RevolutionAngle=180  RevolutionAngleUnits=deg
  sensor4 : sm_lib/Body Elements/Solid  InertiaType=CalculateFromGeometry  Mass=1/1000  MassUnits=kg  CenterOfMass=[0 0 0]  CenterOfMassUnits=m  MomentsOfInertia=[1 1 1]  MomentsOfInertiaUnits=kg*m^2  ProductsOfInertia=[0 0 0]  ProductsOfInertiaUnits=kg*m^2  BasedOnType=Mass  Density=1/1000  DensityUnits=kg/m^3  DoExposeReferenceFrame=on  SerializedFrames=<Frames/>  GraphicType=FromGeometry  MarkerShape=Sphere  MarkerSize=10  GraphicVisPropType=SimpleVisualProperties  GraphicDiffuseColor=[1.0 1.0 0.2]  GraphicSpecularColor=[0.5 0.5 0.5 1.0]  GraphicAmbientColor=[0.15 0.15 0.15 1.0]  GraphicEmissiveColor=[0.0 0.0 0.0 1.0]  GraphicShininess=75  GraphicOpacity=1.0  GeometryShape=Cylinder  RectangleSize=[1 1]  RectangleSizeUnits=m  BrickDimensions=[sensorLength sensorWidth sensorHeight]  BrickDimensionUnits=m  CylinderRadius=sensorSize  CylinderRadiusUnits=m  CylinderLength=sensorHeight  CylinderLengthUnits=m  SphereRadius=1  SphereRadiusUnits=m  EllipsoidRadii=[1 1 .5]  EllipsoidRadiiUnits=m  ExtrusionCrossSection=[1 1; -1 1; -1 -1; 1 -1]  ExtrusionCrossSectionUnits=m  ExtrusionLength=1  ExtrusionLengthUnits=m  PolygonNumSides=3  PolygonOuterRadius=1  PolygonOuterRadiusUnits=m  ExtGeomFileType=STEP  ExtGeomFileName=Bas_assembly_v2.stp  ExtGeomFileUnits=m  RevolutionCrossSection=[1 1; 1 -1; 2 -1; 2 1]  RevolutionCrossSectionUnits=m  RevolutionExtent=Custom  RevolutionAngle=180  RevolutionAngleUnits=deg
  Ground : PMIOPort  Side=Left
  Car Body : PMIOPort  Port=2  Side=Left
  Active1 : Outport
  Active2 : Outport  Port=2
  Active3 : Outport  Port=3
  Active4 : Outport  Port=4
  Active5 : Outport  Port=5
  Active6 : Outport  Port=6
  Active7 : Outport  Port=7
  Active8 : Outport  Port=8
  wires:
  SensorN2/1(Active) -> Active2/1
  SensorN3/1(Active) -> Active3/1
  SensorN4/1(Active) -> Active4/1
  SensorN5/1(Active) -> Active5/1
  SensorN6/1(Active) -> Active6/1
  SensorN7/1(Active) -> Active7/1
  SensorN1/1(Active) -> Active1/1
  SensorN8/1(Active) -> Active8/1
  connections:
  Solid1/RConn1 -- Solid/RConn1 -- Ground/RConn1
  Car Body/RConn1 -- Subsystem2/LConn1 -- Subsystem3/LConn1 -- Subsystem1/LConn1 -- Subsystem8/LConn1 -- Subsystem/LConn1 -- Subsystem5/LConn1 -- Subsystem6/LConn1 -- Subsystem7/LConn1
  SensorN2/LConn1 -- sensor2/RConn1 -- Subsystem1/RConn1
  Subsystem2/RConn1 -- sensor3/RConn1 -- SensorN3/LConn1
  Subsystem3/RConn1 -- sensor4/RConn1 -- SensorN4/LConn1
  Subsystem6/RConn1 -- sensor7/RConn1 -- SensorN7/LConn1
  sensor1/RConn1 -- SensorN1/LConn1 -- Subsystem/RConn1
  SensorN5/LConn1 -- sensor5/RConn1 -- Subsystem8/RConn1
  Subsystem5/RConn1 -- sensor6/RConn1 -- SensorN6/LConn1
  Subsystem7/RConn1 -- sensor8/RConn1 -- SensorN8/LConn1
